simulink model "IdealGen_load_CtrlGen_wDC_abc_detailed"  (R2023b)
settings: Solver=VariableStepAuto  StartTime=0.0  StopTime=Tend  RelTol=1e-3
undefined symbols (not defined in the file): C_dc, C_f, f_nom, H_vsm, Ibase_lv, k_d_vsm, k_p_p_vsm, k_p_q_vsm, Ki_cc, ki_q, Ki_vc, Kp_cc, Kp_vc, l_f, L_f, L_grid, L_mv, l_t_hvmv, l_t_mvlv, Lbase1v, omega_nom, phase_shift_test_state, phase_shifts, Pmax, r_f, R_grid, R_mv, r_t_hvmv, r_t_mvlv, rocof_slope, Rocof_test_state, Sbase1, Sbase_t1, Tchange_gfm_ref, Trocof_end, Trocof_start, V_dc, V_dc_base, Vbase_hv, Vbase_lv, Vbase_mv, voltage_sag_test_state, Zbase1v
libraries: spsControlledVoltageSourceLib x6, slpidlib x5, spsThreePhaseSeriesRLCBranchLib x4, spsPower3phInstantaneousLib x3, spsRMSLib x3, spsabctodq0Lib x3, spsGroundLib x2, spsdq0toabcLib x2, spsCurrentMeasurementLib x2, spsSeriesRLCBranchLib x2, spsVoltageMeasurementLib x2, spsThreePhaseVIMeasurementLib x2
(part 2 of 2)

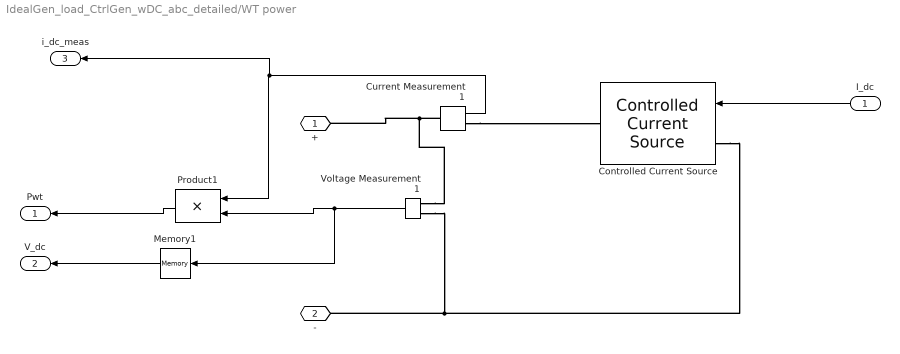
== system IdealGen_load_CtrlGen_wDC_abc_detailed/WT power ==
  I_dc : Inport
  Controlled Current Source : spsControlledCurrentSourceLib/Controlled Current Source  Initialize=on  Source_Type=DC  Amplitude=0  Phase=0  Frequency=0  Measurements=None
  Current Measurement1 : spsCurrentMeasurementLib/Current Measurement  PhasorSimulation=off  OutputType=Complex  PSBequivalent=0
  Memory1 : Memory  InitialCondition=V_dc
  Product1 : Product  SaturateOnIntegerOverflow=on  OutDataTypeStr=Inherit: Same as first input
  Voltage Measurement1 : spsVoltageMeasurementLib/Voltage Measurement  PhasorSimulation=off  OutputType=Complex  PSBequivalent=0
  + : PMIOPort  Side=Right
  - : PMIOPort  Port=2  Side=Right
  Pwt : Outport
  V_dc : Outport  Port=2
  i_dc_meas : Outport  Port=3
  wires:
  Current Measurement1/1 -> i_dc_meas/1, Product1/1
  Product1/1 -> Pwt/1
  Voltage Measurement1/1 -> Memory1/1, Product1/2
  I_dc/1 -> Controlled Current Source/1
  Memory1/1 -> V_dc/1
  connections:
  Controlled Current Source/LConn1 -- Voltage Measurement1/LConn2 -- -/RConn1
  Current Measurement1/LConn1 -- Voltage Measurement1/LConn1 -- +/RConn1
  Current Measurement1/RConn1 -- Controlled Current Source/RConn1

== system IdealGen_load_CtrlGen_wDC_abc_detailed/constant DC Voltage ==
  DC Voltage Source2 : spsDCVoltageSourceLib/DC Voltage Source  Amplitude=V_dc/2  Measurements=None
  DC Voltage Source3 : spsDCVoltageSourceLib/DC Voltage Source  Amplitude=V_dc/2  Measurements=None
  + : PMIOPort  Side=Left
  - : PMIOPort  Port=2  Side=Right
  connections:
  DC Voltage Source2/LConn1 -- DC Voltage Source3/RConn1
  DC Voltage Source2/RConn1 -- +/RConn1
  DC Voltage Source3/LConn1 -- -/RConn1

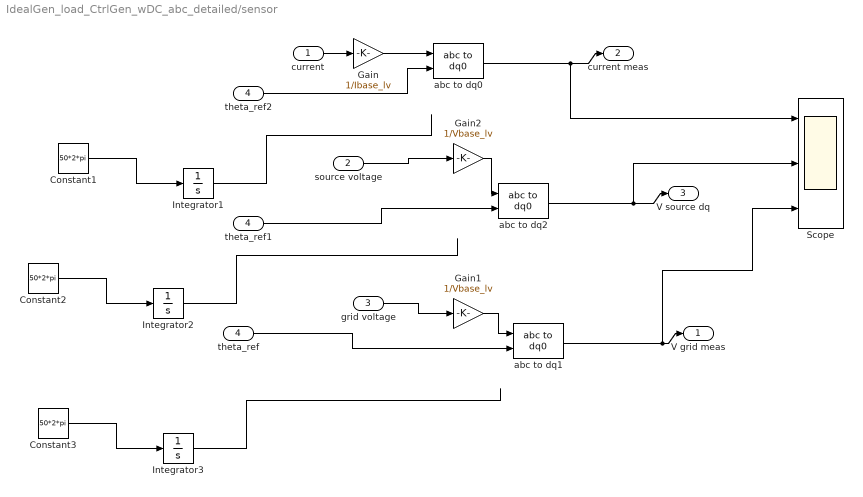
== system IdealGen_load_CtrlGen_wDC_abc_detailed/sensor ==
  current : Inport
  source voltage : Inport  Port=2
  grid voltage : Inport  Port=3
  theta_ref : Inport  Port=4
  Constant1 : Constant  Value=50*2*pi
  Constant2 : Constant  Value=50*2*pi
  Constant3 : Constant  Value=50*2*pi
  Gain : Gain  Gain=1/Ibase_lv
  Gain1 : Gain  Gain=1/Vbase_lv
  Gain2 : Gain  Gain=1/Vbase_lv
  Integrator1 : Integrator
  Integrator2 : Integrator
  Integrator3 : Integrator
  Scope : Scope  NumInputPorts=3
  abc to dq0 : spsabctodq0Lib/abc to dq0  Alignment=90 degrees behind phase A axis
  abc to dq1 : spsabctodq0Lib/abc to dq0  Alignment=90 degrees behind phase A axis
  abc to dq2 : spsabctodq0Lib/abc to dq0  Alignment=90 degrees behind phase A axis
  theta_ref1 : InportShadow  Port=4
  theta_ref2 : InportShadow  Port=4
  V grid meas : Outport
  current meas : Outport  Port=2
  V source dq : Outport  Port=3
  wires:
  Gain/1 -> abc to dq0/1
  abc to dq0/1 -> Scope/1, current meas/1
  abc to dq1/1 -> Scope/3, V grid meas/1
  grid voltage/1 -> Gain1/1
  source voltage/1 -> Gain2/1
  abc to dq2/1 -> Scope/2, V source dq/1
  Integrator1/1 -> ?
  Constant1/1 -> Integrator1/1
  theta_ref/1 -> abc to dq1/2
  theta_ref1/1 -> abc to dq2/2
  theta_ref2/1 -> abc to dq0/2
  Constant2/1 -> Integrator2/1
  Integrator2/1 -> ?
  Integrator3/1 -> ?
  Constant3/1 -> Integrator3/1
  Gain2/1 -> abc to dq2/1
  current/1 -> Gain/1
  Gain1/1 -> abc to dq1/1
